simulink model "TwoMassComObservadorKalman"  (R2024b)
settings: Solver=VariableStepAuto  StartTime=0.0  StopTime=10  MaxStep=0.01  RelTol=1e-3
values from neighbouring files (symbols this model uses):
  KL = lqr(Aol,Bol,Q,R)    [TwoMassModel.m]
  N1 = -inv(C1*inv(Aol-Bol*KL)*Bol)    [TwoMassModel.m]
libraries: cstblocks x5
settings Model: Creator=jorgeferreira  LastModifiedBy=jorgeferreira
settings DebuggingCC: UnconnectedInputMsg=warning  UnconnectedOutputMsg=warning  UnconnectedLineMsg=warning
settings ModelReferenceCC: EnableRefExpFcnMdlSchedulingChecks=on
settings RTWCC: GPUComputeCapability=3.5  DLArmComputeVersion=19.05

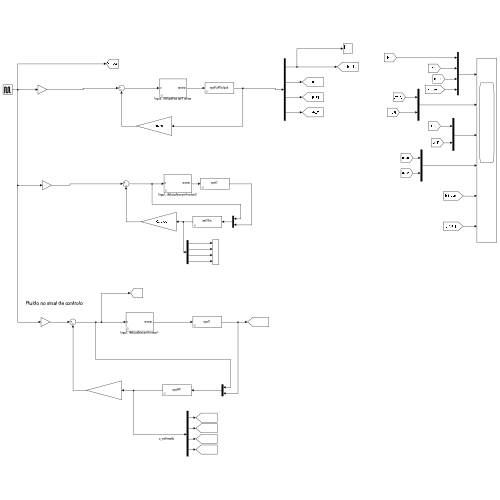
[thumbnail: Simulink's stored preview of the top-level diagram]
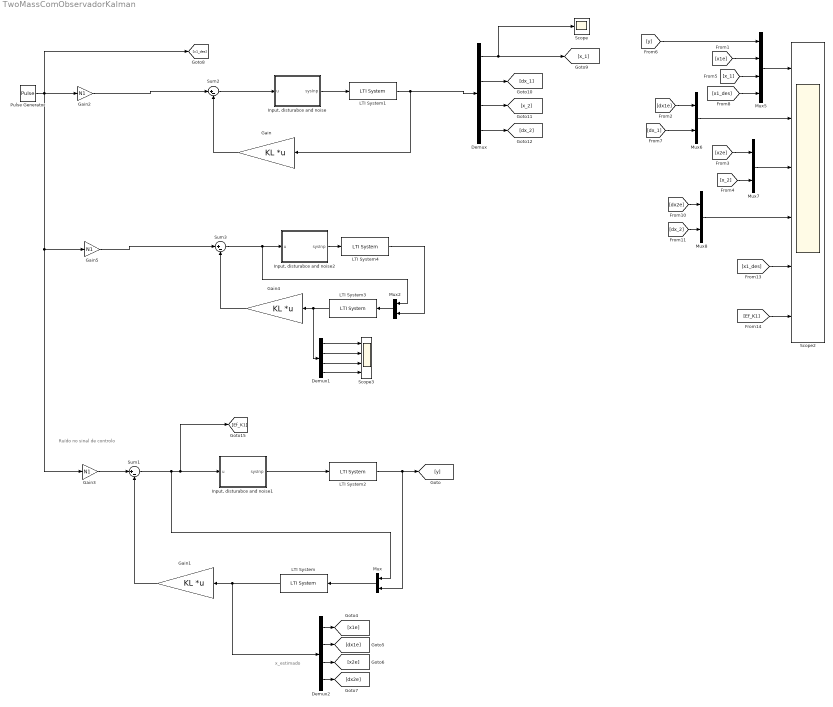
== system TwoMassComObservadorKalman ==
  note: Ruído no sinal de controlo
  note: x_estimado
  Demux : Demux
  Demux1 : Demux
  Demux2 : Demux
  Gain : Gain  Gain=KL  Multiplication=Matrix(K*u) (u vector)
  Gain1 : Gain  Gain=KL  Multiplication=Matrix(K*u) (u vector)
  Gain2 : Gain  Gain=N1
  Gain3 : Gain  Gain=N1
  Gain4 : Gain  Gain=KL  Multiplication=Matrix(K*u) (u vector)
  Gain5 : Gain  Gain=N1
  "Input, disturabce and noise" : Subsystem  mask{noiseVar=0.1}
      mask prompts: noiseVar "Noise variance"
  "Input, disturabce and noise1" : Subsystem  mask{noiseVar=0.1}
      mask prompts: noiseVar "Noise variance"
  "Input, disturabce and noise2" : Subsystem  mask{noiseVar=0}
      mask prompts: noiseVar "Noise variance"
  LTI System : cstblocks/LTI System  sys=sysKF  IC=x0  PadeOrder=0
  LTI System1 : cstblocks/LTI System  sys=sysFullOutput  IC=x0  PadeOrder=0
  LTI System2 : cstblocks/LTI System  sys=sysC  IC=x0  PadeOrder=0
  LTI System3 : cstblocks/LTI System  sys=esObs  IC=x0  PadeOrder=0
  LTI System4 : cstblocks/LTI System  sys=sysC  IC=x0  PadeOrder=0
  Mux{,2,6..8} (5 alike) : Mux  Inputs=2
  Mux5 : Mux
  Pulse Generator : DiscretePulseGenerator  PulseType=Time based  Period=5  PulseWidth=50  PhaseDelay=2
  Scope : Scope
  Scope2 : Scope  NumInputPorts=6
  Scope3 : Scope  NumInputPorts=4
  Sum1 : Sum  Inputs=|+-
  Sum2 : Sum  Inputs=|+-
  Sum3 : Sum  Inputs=|+-
  wires:
  Mux/1 -> LTI System/1
  Mux5/1 -> Scope2/1
  Mux6/1 -> Scope2/2
  Demux2/1 -> [x1e]
  Demux2/2 -> [dx1e]
  Demux2/3 -> [x2e]
  Demux2/4 -> [dx2e]
  Demux/4 -> [dx_2]
  Demux/3 -> [x_2]
  Demux/2 -> [dx_1]
  Demux/1 -> Scope/1, [x_1]
  Mux7/1 -> Scope2/3
  [dx_2] -> Mux8/2
  Mux8/1 -> Scope2/4
  [x1_des] -> Scope2/5
  [Ef_K1] -> Scope2/6
  LTI System1/1 -> Gain/1, Demux/1
  LTI System/1 -> Demux2/1, Gain1/1
  "Input, disturabce and noise"/1(sysInp) -> LTI System1/1
  "Input, disturabce and noise1"/1(sysInp) -> LTI System2/1
  LTI System2/1 -> [y], Mux/2
  [x_1] -> Mux5/3
  [x1e] -> Mux5/2
  [y] -> Mux5/1
  Sum1/1 -> Mux/1, [Ef_K1], "Input, disturabce and noise1"/1(u)
  Gain1/1 -> Sum1/2
  Gain/1 -> Sum2/2
  Sum2/1 -> "Input, disturabce and noise"/1(u)
  [dx1e] -> Mux6/1
  [dx_1] -> Mux6/2
  [dx2e] -> Mux8/1
  [x2e] -> Mux7/1
  [x_2] -> Mux7/2
  Gain3/1 -> Sum1/1
  [x1_des] -> Mux5/4
  Gain4/1 -> Sum3/2
  Pulse Generator/1 -> [x1_des], Gain5/1, Gain3/1, Gain2/1
  Gain5/1 -> Sum3/1
  Sum3/1 -> Mux2/1, "Input, disturabce and noise2"/1(u)
  LTI System3/1 -> Demux1/1, Gain4/1
  "Input, disturabce and noise2"/1(sysInp) -> LTI System4/1
  LTI System4/1 -> Mux2/2
  Mux2/1 -> LTI System3/1
  Demux1/1 -> Scope3/1
  Demux1/2 -> Scope3/2
  Demux1/3 -> Scope3/3
  Demux1/4 -> Scope3/4
  Gain2/1 -> Sum2/1

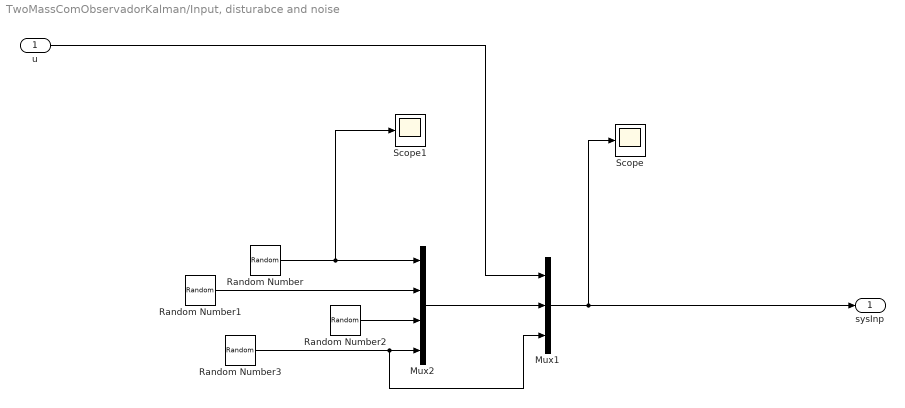
== system TwoMassComObservadorKalman/Input, disturabce and noise ==
  u : Inport
  Mux1 : Mux  Inputs=3
  Mux2 : Mux
  Random Number{,1..3} (4 alike) : RandomNumber  Variance=noiseVar  SampleTime=0.02
  Scope : Scope
  Scope1 : Scope
  sysInp : Outport
  wires:
  Random Number1/1 -> Mux2/2
  Mux1/1 -> Scope/1, sysInp/1
  Random Number2/1 -> Mux2/3
  Random Number3/1 -> Mux1/3, Mux2/4
  Mux2/1 -> Mux1/2
  u/1 -> Mux1/1
  Random Number/1 -> Scope1/1, Mux2/1

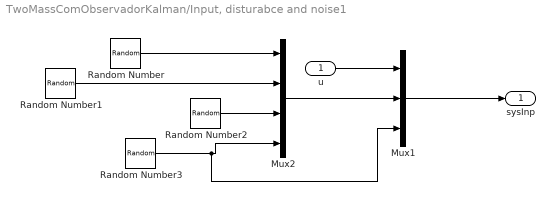
== system TwoMassComObservadorKalman/Input, disturabce and noise1 ==
  u : Inport
  Mux1 : Mux  Inputs=3
  Mux2 : Mux
  Random Number{,1..3} (4 alike) : RandomNumber  Variance=noiseVar  SampleTime=0.02
  sysInp : Outport
  wires:
  Random Number/1 -> Mux2/1
  u/1 -> Mux1/1
  Mux2/1 -> Mux1/2
  Random Number3/1 -> Mux2/4, Mux1/3
  Random Number2/1 -> Mux2/3
  Mux1/1 -> sysInp/1
  Random Number1/1 -> Mux2/2

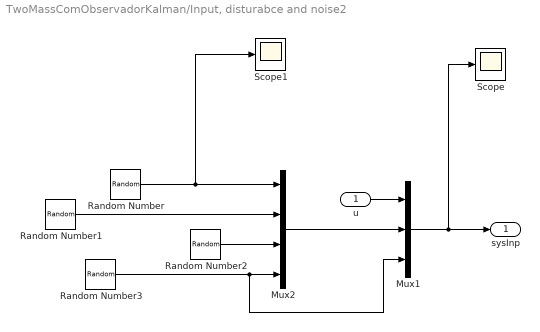
== system TwoMassComObservadorKalman/Input, disturabce and noise2 ==
  u : Inport
  Mux1 : Mux  Inputs=3
  Mux2 : Mux
  Random Number{,1..3} (4 alike) : RandomNumber  Variance=noiseVar  SampleTime=0.02
  Scope : Scope
  Scope1 : Scope
  sysInp : Outport
  wires:
  Random Number1/1 -> Mux2/2
  Mux1/1 -> Scope/1, sysInp/1
  Random Number2/1 -> Mux2/3
  Random Number3/1 -> Mux1/3, Mux2/4
  Mux2/1 -> Mux1/2
  u/1 -> Mux1/1
  Random Number/1 -> Scope1/1, Mux2/1
